simulink model "Quad_PID_FUSION"  (R2023b)
settings: Solver=ode1  StartTime=0.0  StopTime=200  FixedStep=0.01  RelTol=1e-3
values from neighbouring files (symbols this model uses):
  Quad_Model = struct(     'Ixx', 0.016,      'Iyy', 0.016,      'Izz', 0.0274,      'Im', 3.789e-6,      'mass', 1,      'g', 9.8)    [Quad_PID_FUSION_Pipeline.m]    (also in Quad_PID_FUSION_Pipeline_Close_Loop_Attack.m; Quad_PID_FUSION_Pipeline_Close_Loop_Attack_Pipeline.m; Quad_PID_FUSION_Pipeline_Close_Loop_Attack_Pipeline_Reach.m; Quad_PID_FUSION_Pipeline_Close_Loop_Attack_Pipeline_Repeat_V5.m)
  s_x_0 = 0.0    (= 0)    [Quad_PID_FUSION_Pipeline.m]    (also in Quad_PID_FUSION_Pipeline_Loop_Attack_Execution.m = current_norm * cos(angle))
  s_y_0 = 0.0    (= 0)    [Quad_PID_FUSION_Pipeline.m]    (also in Quad_PID_FUSION_Pipeline_Loop_Attack_Execution.m = current_norm * sin(angle))
undefined symbols (not defined in the file or in its folder): DiscIntNeverNeededParam
libraries: simulink x9
(part 2 of 2)

== matlab function Quad_PID_FUSION/Position Controller/MATLAB Function ==
  data: thrust_x input; thrust_sp_x output; thrust_y input; thrust_z input; thrust_sp_y output; thtust_sp_z output
function [thrust_sp_x,thrust_sp_y,thtust_sp_z] = Thrust_Limit(thrust_x,thrust_y,thrust_z)

MPC_THR_MIN = 0.1;
MPC_THR_MAX = 0.9;
tilt_max = 20;

thtust_sp_z = constrain_function2( thrust_z, MPC_THR_MIN, MPC_THR_MAX);

thrust_max_XY_tilt = abs(thtust_sp_z) * tan(tilt_max/180.0*pi);
thrust_max_XY = sqrt(MPC_THR_MAX * MPC_THR_MAX - thtust_sp_z * thtust_sp_z);

thrust_max_XY = min(thrust_max_XY_tilt, thrust_max_XY);


if (thrust_x^2 + thrust_y^2) > thrust_max_XY^2 
    mag = sqrt(thrust_x^2 + thrust_y^2);
    thrust_sp_x = thrust_x / mag * thrust_max_XY;
    thrust_sp_y = thrust_y / mag * thrust_max_XY;
else
    thrust_sp_x = thrust_x;
    thrust_sp_y = thrust_y;
end

end
function output = constrain_function2(data, Min, Max)
    
    if data > Max
        output =  Max;
    elseif data < Min
        output = Min;
    else
        output = data;
    end
end

== matlab function Quad_PID_FUSION/thrust_to_motor_speed ==
  data: w_1 output; torque_x input; torque_y input; w_2 output; torque_z input; thrust input; w_3 output; w_4 output
function [w_1, w_2, w_3, w_4] = thrust_to_motor_speed(torque_x, torque_y, torque_z, thrust)


w_1 = 0;
w_2 = 0;
w_3 = 0;
w_4 = 0;

d  = 0.2;
cT_est = 1.239e-5;
cM_est = 1.982e-7;


M4 = [-sqrt(2)/2*d*cT_est,sqrt(2)/2*d*cT_est,sqrt(2)/2*d*cT_est,-sqrt(2)/2*d*cT_est;
       sqrt(2)/2*d*cT_est,-sqrt(2)/2*d*cT_est,sqrt(2)/2*d*cT_est,-sqrt(2)/2*d*cT_est;
       cM_est,cM_est,-cM_est,-cM_est;
       cT_est,cT_est,cT_est,cT_est;];

w =  M4 \ [torque_x;torque_y;torque_z;thrust];

% w_1 = sqrt(w(1));
% w_2 = sqrt(w(2));
% w_3 = sqrt(w(3));
% w_4 = sqrt(w(4));

w_1 = sqrt(max([0,w(1)]));
w_2 = sqrt(max([0,w(2)]));
w_3 = sqrt(max([0,w(3)]));
w_4 = sqrt(max([0,w(4)]));


end

== matlab function Quad_PID_FUSION/GPS ==
  settings: updateMethod=DISCRETE
  data: local_pos_gps output; pos_x input; pos_y input; pos_z input; vel_x input; vel_gps output; vel_y input; vel_z input
function [local_pos_gps, vel_gps] = GPS2LLA2GPS(pos_x, pos_y, pos_z, vel_x, vel_y, vel_z)

%GPS
gpsFs = 1;
% GPS = gpsSensor('UpdateRate', gpsFs);
GPS = gpsSensor('ReferenceFrame','NED','SampleRate',gpsFs);
GPS.HorizontalPositionAccuracy = 1;
GPS.VerticalPositionAccuracy = 1;
GPS.VelocityAccuracy = 0.1;
% [lla_pos,lla_vel] = GPS([pos(1),pos(2),pos(3)], [vel(1),vel(2),vel(3)]);
[lla_pos,lla_vel] = GPS([pos_x,pos_y,pos_z], [vel_x,vel_y,vel_z]);
lla0 = [0, 0, 0];
method = 'flat';
local_pos_gps = lla2ned(lla_pos,lla0,method);
vel_gps = lla_vel;
